simulink model "actividad2simulink"  (R2021a)
settings: Solver=ode1  StartTime=0.0  StopTime=10.0  FixedStep=0.001  RelTol=1e-3
values from neighbouring files (symbols this model uses):
  C = 18e-6    (= 1.8e-05)    [actividad2.m]
  R = 10000    [actividad2.m]
settings Model: Creator=Agus  LastModifiedBy=Agus

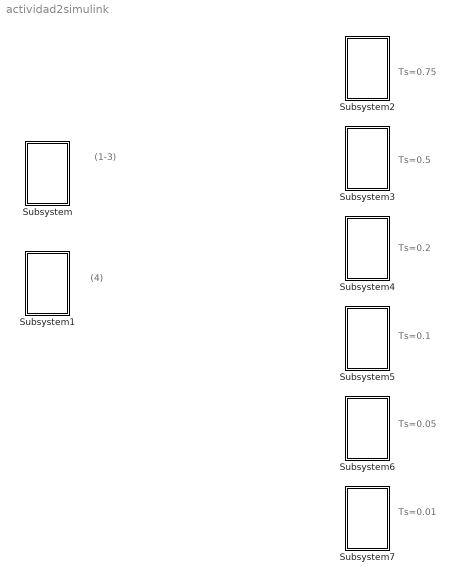
== system actividad2simulink ==
  note: Ts=0.75
  note: (4)
  note: (1-3)
  note: Ts=0.5
  note: Ts=0.2
  note: Ts=0.1
  note: Ts=0.05
  note: Ts=0.01
  Subsystem : Subsystem
  Subsystem1 : Subsystem
  Subsystem2 : Subsystem
  Subsystem3 : Subsystem
  Subsystem4 : Subsystem
  Subsystem5 : Subsystem
  Subsystem6 : Subsystem
  Subsystem7 : Subsystem

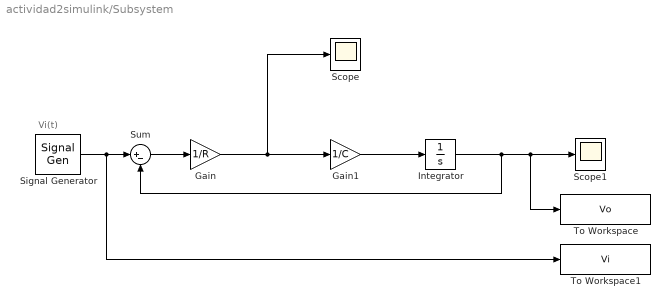
== system actividad2simulink/Subsystem ==
  note: Vi(t)
  Gain : Gain  Gain=1/R
  Gain1 : Gain  Gain=1/C
  Integrator : Integrator
  Scope : Scope
  Scope1 : Scope
  Signal Generator : SignalGenerator  Amplitude=2.5
  Sum : Sum  Inputs=|+-
  To Workspace : ToWorkspace  VariableName=Vo  SaveFormat=Timeseries  SampleTime=-1
  To Workspace1 : ToWorkspace  VariableName=Vi  SaveFormat=Timeseries  SampleTime=-1
  wires:
  Signal Generator/1 -> To Workspace1/1, Sum/1
  Gain/1 -> Scope/1, Gain1/1
  Integrator/1 -> Sum/2, To Workspace/1, Scope1/1
  Sum/1 -> Gain/1
  Gain1/1 -> Integrator/1

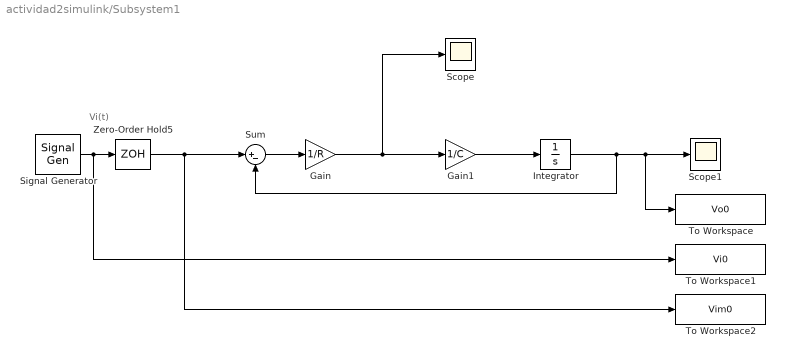
== system actividad2simulink/Subsystem1 ==
  note: Vi(t)
  Gain : Gain  Gain=1/R
  Gain1 : Gain  Gain=1/C
  Integrator : Integrator
  Scope : Scope
  Scope1 : Scope
  Signal Generator : SignalGenerator  Amplitude=2.5
  Sum : Sum  Inputs=|+-
  To Workspace : ToWorkspace  VariableName=Vo0  SaveFormat=Timeseries  SampleTime=-1
  To Workspace1 : ToWorkspace  VariableName=Vi0  SaveFormat=Timeseries  SampleTime=-1
  To Workspace2 : ToWorkspace  VariableName=Vim0  SampleTime=-1
  Zero-Order Hold5 : ZeroOrderHold  SampleTime=0.75
  wires:
  Gain/1 -> Scope/1, Gain1/1
  Integrator/1 -> Sum/2, To Workspace/1, Scope1/1
  Sum/1 -> Gain/1
  Gain1/1 -> Integrator/1
  Signal Generator/1 -> To Workspace1/1, Zero-Order Hold5/1
  Zero-Order Hold5/1 -> To Workspace2/1, Sum/1

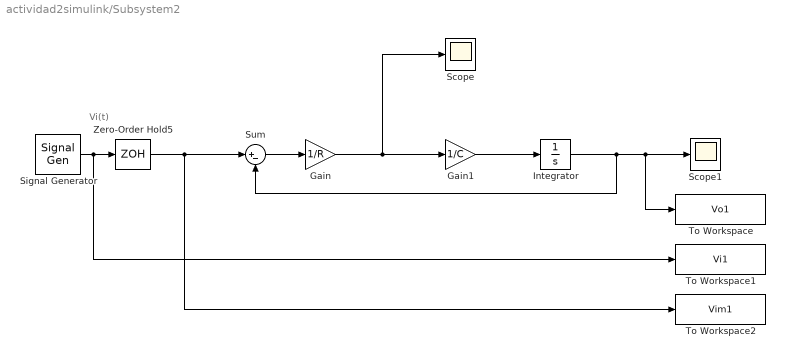
== system actividad2simulink/Subsystem2 ==
  note: Vi(t)
  Gain : Gain  Gain=1/R
  Gain1 : Gain  Gain=1/C
  Integrator : Integrator
  Scope : Scope
  Scope1 : Scope
  Signal Generator : SignalGenerator  Amplitude=2.5
  Sum : Sum  Inputs=|+-
  To Workspace : ToWorkspace  VariableName=Vo1  SaveFormat=Timeseries  SampleTime=-1
  To Workspace1 : ToWorkspace  VariableName=Vi1  SaveFormat=Timeseries  SampleTime=-1
  To Workspace2 : ToWorkspace  VariableName=Vim1  SaveFormat=Timeseries  SampleTime=-1
  Zero-Order Hold5 : ZeroOrderHold  SampleTime=0.75
  wires:
  Gain/1 -> Scope/1, Gain1/1
  Integrator/1 -> Sum/2, To Workspace/1, Scope1/1
  Sum/1 -> Gain/1
  Gain1/1 -> Integrator/1
  Signal Generator/1 -> To Workspace1/1, Zero-Order Hold5/1
  Zero-Order Hold5/1 -> To Workspace2/1, Sum/1

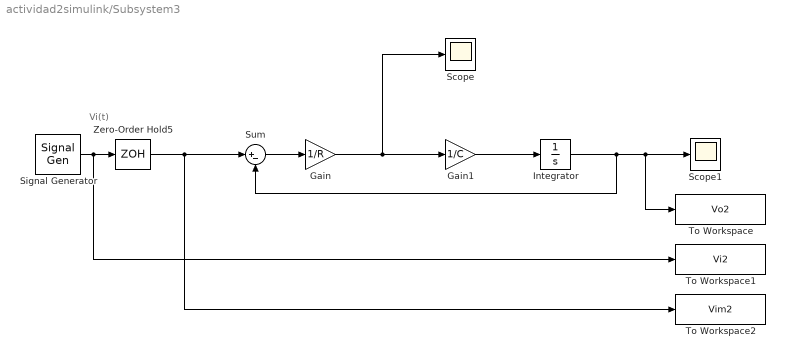
== system actividad2simulink/Subsystem3 ==
  note: Vi(t)
  Gain : Gain  Gain=1/R
  Gain1 : Gain  Gain=1/C
  Integrator : Integrator
  Scope : Scope
  Scope1 : Scope
  Signal Generator : SignalGenerator  Amplitude=2.5
  Sum : Sum  Inputs=|+-
  To Workspace : ToWorkspace  VariableName=Vo2  SaveFormat=Timeseries  SampleTime=-1
  To Workspace1 : ToWorkspace  VariableName=Vi2  SaveFormat=Timeseries  SampleTime=-1
  To Workspace2 : ToWorkspace  VariableName=Vim2  SaveFormat=Timeseries  SampleTime=-1
  Zero-Order Hold5 : ZeroOrderHold  SampleTime=0.5
  wires:
  Gain/1 -> Scope/1, Gain1/1
  Integrator/1 -> Sum/2, To Workspace/1, Scope1/1
  Sum/1 -> Gain/1
  Gain1/1 -> Integrator/1
  Signal Generator/1 -> To Workspace1/1, Zero-Order Hold5/1
  Zero-Order Hold5/1 -> To Workspace2/1, Sum/1

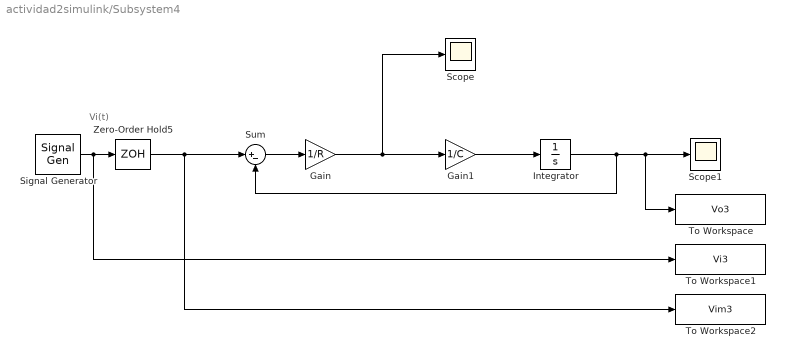
== system actividad2simulink/Subsystem4 ==
  note: Vi(t)
  Gain : Gain  Gain=1/R
  Gain1 : Gain  Gain=1/C
  Integrator : Integrator
  Scope : Scope
  Scope1 : Scope
  Signal Generator : SignalGenerator  Amplitude=2.5
  Sum : Sum  Inputs=|+-
  To Workspace : ToWorkspace  VariableName=Vo3  SaveFormat=Timeseries  SampleTime=-1
  To Workspace1 : ToWorkspace  VariableName=Vi3  SaveFormat=Timeseries  SampleTime=-1
  To Workspace2 : ToWorkspace  VariableName=Vim3  SaveFormat=Timeseries  SampleTime=-1
  Zero-Order Hold5 : ZeroOrderHold  SampleTime=0.2
  wires:
  Gain/1 -> Scope/1, Gain1/1
  Integrator/1 -> Sum/2, To Workspace/1, Scope1/1
  Sum/1 -> Gain/1
  Gain1/1 -> Integrator/1
  Signal Generator/1 -> To Workspace1/1, Zero-Order Hold5/1
  Zero-Order Hold5/1 -> To Workspace2/1, Sum/1

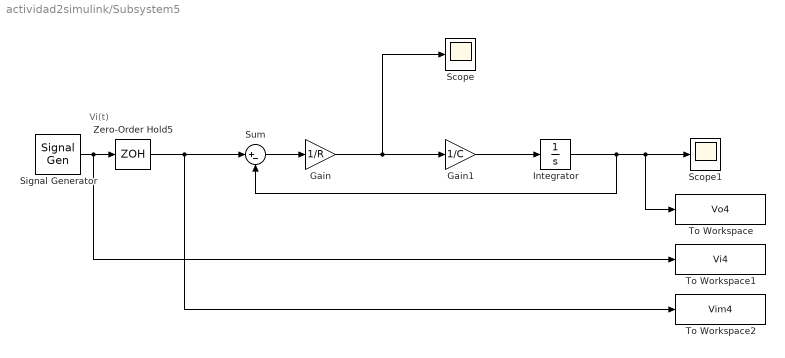
== system actividad2simulink/Subsystem5 ==
  note: Vi(t)
  Gain : Gain  Gain=1/R
  Gain1 : Gain  Gain=1/C
  Integrator : Integrator
  Scope : Scope
  Scope1 : Scope
  Signal Generator : SignalGenerator  Amplitude=2.5
  Sum : Sum  Inputs=|+-
  To Workspace : ToWorkspace  VariableName=Vo4  SaveFormat=Timeseries  SampleTime=-1
  To Workspace1 : ToWorkspace  VariableName=Vi4  SaveFormat=Timeseries  SampleTime=-1
  To Workspace2 : ToWorkspace  VariableName=Vim4  SaveFormat=Timeseries  SampleTime=-1
  Zero-Order Hold5 : ZeroOrderHold  SampleTime=0.1
  wires:
  Gain/1 -> Scope/1, Gain1/1
  Integrator/1 -> Sum/2, To Workspace/1, Scope1/1
  Sum/1 -> Gain/1
  Gain1/1 -> Integrator/1
  Signal Generator/1 -> To Workspace1/1, Zero-Order Hold5/1
  Zero-Order Hold5/1 -> To Workspace2/1, Sum/1

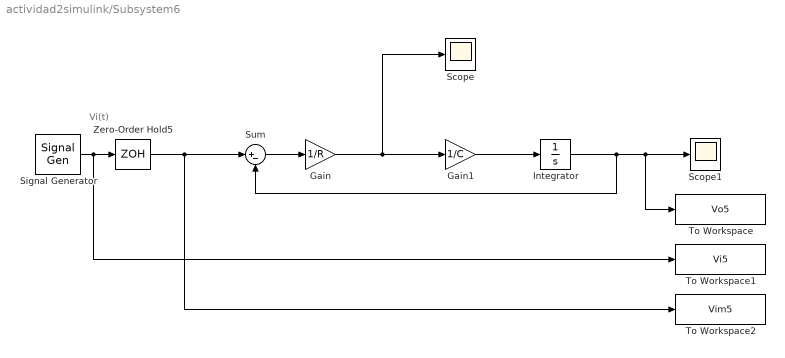
== system actividad2simulink/Subsystem6 ==
  note: Vi(t)
  Gain : Gain  Gain=1/R
  Gain1 : Gain  Gain=1/C
  Integrator : Integrator
  Scope : Scope
  Scope1 : Scope
  Signal Generator : SignalGenerator  Amplitude=2.5
  Sum : Sum  Inputs=|+-
  To Workspace : ToWorkspace  VariableName=Vo5  SaveFormat=Timeseries  SampleTime=-1
  To Workspace1 : ToWorkspace  VariableName=Vi5  SaveFormat=Timeseries  SampleTime=-1
  To Workspace2 : ToWorkspace  VariableName=Vim5  SaveFormat=Timeseries  SampleTime=-1
  Zero-Order Hold5 : ZeroOrderHold  SampleTime=0.05
  wires:
  Gain/1 -> Scope/1, Gain1/1
  Integrator/1 -> Sum/2, To Workspace/1, Scope1/1
  Sum/1 -> Gain/1
  Gain1/1 -> Integrator/1
  Signal Generator/1 -> To Workspace1/1, Zero-Order Hold5/1
  Zero-Order Hold5/1 -> To Workspace2/1, Sum/1

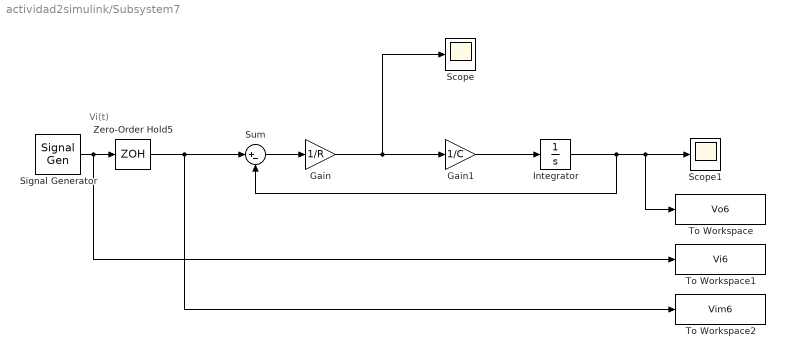
== system actividad2simulink/Subsystem7 ==
  note: Vi(t)
  Gain : Gain  Gain=1/R
  Gain1 : Gain  Gain=1/C
  Integrator : Integrator
  Scope : Scope
  Scope1 : Scope
  Signal Generator : SignalGenerator  Amplitude=2.5
  Sum : Sum  Inputs=|+-
  To Workspace : ToWorkspace  VariableName=Vo6  SaveFormat=Timeseries  SampleTime=-1
  To Workspace1 : ToWorkspace  VariableName=Vi6  SaveFormat=Timeseries  SampleTime=-1
  To Workspace2 : ToWorkspace  VariableName=Vim6  SaveFormat=Timeseries  SampleTime=-1
  Zero-Order Hold5 : ZeroOrderHold  SampleTime=0.01
  wires:
  Gain/1 -> Scope/1, Gain1/1
  Integrator/1 -> Sum/2, To Workspace/1, Scope1/1
  Sum/1 -> Gain/1
  Gain1/1 -> Integrator/1
  Signal Generator/1 -> To Workspace1/1, Zero-Order Hold5/1
  Zero-Order Hold5/1 -> To Workspace2/1, Sum/1
